simulink model "TorqueSpeedCharOf3phaseIM"  (R2021a)
settings: Solver=VariableStepAuto  StartTime=0.0  StopTime=10.0  RelTol=1e-3
libraries: simulink x2, spsAsynchronousMachineSIUnitsLib x1, spsSampleandHoldLib x1, spsThreePhaseSourceLib x1, spspowerguiLib x1
settings Model: Creator=nabaj  LastModifiedBy=nabaj

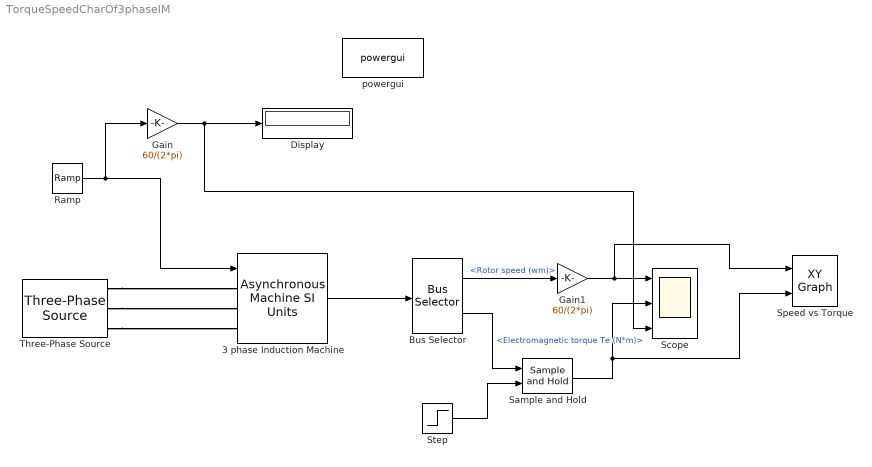
== system TorqueSpeedCharOf3phaseIM ==
  3 phase Induction Machine : spsAsynchronousMachineSIUnitsLib/Asynchronous Machine SI Units  RotorType=Squirrel-cage  PresetModel="15:  5.4 HP (4KW)   400 V  50Hz 1430 RPM"  MechanicalLoad=Speed w  ShowDetailedParameters=on  ReferenceFrame=Stationary  Units=SI  MeasurementBus=off  NominalParameters=[4000 400 50]  VoltageRatio=1  Stator=[1.405 0.005839]  Rotor=[1.395 0.005839]  Cage1=[0.4155 0.002066]  Cage2=[0.4168 0.0003495]  Lm=0.1722  Mechanical=[0.0131 0.002985 2]  PolePairs=2  InitialConditions=[0 0 0 0 0 0 0 0]  SimulateSaturation=off  Saturation=[14.03593122, 27.81365428, 53.79336849, 72.68890987, 97.98006896, 148.6815601, 215.7428561, 302.9841135, 428.7778367 ; 230, 322, 414, 460, 506, 552, 598, 644, 690]  LoadFlowParameters=1492000  TsPowergui=0  TsBlock=-1  IterativeModel=Trapezoidal non iterative  IterativeDiscreteModel=Trapezoidal non iterative  Pmec=1.492e+006
  Bus Selector : BusSelector  OutputSignals=Mechanical.Rotor speed (wm),Mechanical.Electromagnetic torque Te (N*m)
  Display : Display
  Gain : Gain  Gain=60/(2*pi)
  Gain1 : Gain  Gain=60/(2*pi)
  Ramp : simulink/Sources/Ramp  slope=16  start=0  InitialOutput=0
  Sample and Hold : spsSampleandHoldLib/Sample and Hold  ic=70  Ts=0
      settings: SourceProductBaseCode=PS
  Scope : Scope  NumInputPorts=3
  Speed vs Torque : simulink/Sinks/XY Graph  xmin=0  xmax=1500  ymin=0  ymax=100  st=0.5
  Step : Step  SampleTime=0
  Three-Phase Source : spsThreePhaseSourceLib/Three-Phase Source  InternalConnection=Yg  VoltagePhases=off  Voltage=400  PhaseAngle=0  Voltage_phases=[25e3 25e3 25e3]/sqrt(3)  PhaseAngles_phases=[0 -120 +120]  Frequency=50  NonIdealSource=off  SpecifyImpedance=off  Resistance=0.8929  Inductance=16.58e-3  ShortCircuitLevel=100e6  BaseVoltage=25e3  XRratio=7  BusType=swing  Pref=10e3  Qref=0  Prefabc=[10e3, 10e3, 10e3]  Qrefabc=[0, 0, 0]  Qmin=-inf  Qmax=inf
  powergui : spspowerguiLib/powergui  Priority=1  SimulationMode=Continuous  SampleTime=50e-6  frequency=60  Iterations=50  frequencyindice=50  Pbase=100e6  ErrMax=1e-4  UnitsV=kV  UnitsW=MW  buscounter=0  FunctionMessages=off  echomessages=off  EnableUseOfTLC=off  CurrentSourceSwitches=off  DisableSnubberDevices=off  DisableRonSwitches=off  DisableVfSwitches=off  DisplayEquations=off  AutomaticDiscreteSolvers=off  SolverType=Tustin/Backward Euler (TBE)  Interpol=off  ExternalGateDelay=off  methode=off  Ts=100  x0status=blocks  SPID=on  SwTol=0  HookPort=off  NonlinearTolerance=1e-4  nMaxIteration=100  ContinueOnMaxIteration=off  RestoreLinks=warning  ResistiveCurrentMeasurement=off  Frange=[0:2:500]  Ylog=off  Xlog=on  ShowGrid=off  save=off  variable=ZData  structure=0  ZoomFFT=off  StartTime=0.0  cycles=1  DisplayStyle=1  fundamental=60  FreqAxis=off  MaxFrequency=1000  frequencyindicesteady=1  RmsSteady=1  display=off
  wires:
  Ramp/1 -> Gain/1, 3 phase Induction Machine/1
  Gain/1 -> Scope/3, Display/1
  3 phase Induction Machine/1 -> Bus Selector/1
  Bus Selector/1 -> Gain1/1  "<Rotor speed (wm)>"
  Gain1/1 -> Speed vs Torque/1, Scope/1
  Bus Selector/2 -> Sample and Hold/1  "<Electromagnetic torque Te (N*m)>"
  Step/1 -> Sample and Hold/2
  Sample and Hold/1 -> Speed vs Torque/2, Scope/2
  connections:
  Three-Phase Source/RConn1 -- 3 phase Induction Machine/LConn1
  Three-Phase Source/RConn2 -- 3 phase Induction Machine/LConn2
  Three-Phase Source/RConn3 -- 3 phase Induction Machine/LConn3
